simulink model "unfinished_Test_Display"  (Simulink 8.1)
settings: Solver=ode45  SolverMode=SingleTasking  StartTime=0.0  StopTime=2  RelTol=1e-3
undefined symbols (not defined in the file): A, ARROW_DOWN, ARROW_LEFT, ARROW_RIGHT, ARROW_UP, ASTERISK, B, BACKSLASH, C, COLON, COMMA, CROSS, CURSOR, D, DOT, EQUAL, EXCLAMATION_MARK, F, G, GREATER_THAN, H, HEIGHT, hot, I, J, K, L, LEFT_PARENTHESES, LESS_THAN, M, MINUS, N, O, P, PERCENT, PLUS, POS_X, POS_Y, Q, QUESTION_MARK, QUOTE, R, RECTANGLE, RIGHT_PARENTHESES, S, SEMICOLON, SHARP, SLASH, SPACE, T, U, UNDERSCORE, V, vect, W, WIDTH, X, Y, Z, ZERO
libraries: Common_Library x40, dspsnks4 x2, commutil2 x1
(part 2 of 3)

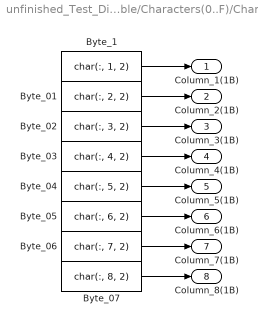
== system unfinished_Test_Display/Character_Table/Characters(0..F)/Char_2 ==
  Byte_01 : Constant  Value=char(:, 2, 2)  OutDataTypeStr=uint8
  Byte_02 : Constant  Value=char(:, 3, 2)  OutDataTypeStr=uint8
  Byte_03 : Constant  Value=char(:, 4, 2)  OutDataTypeStr=uint8
  Byte_04 : Constant  Value=char(:, 5, 2)  OutDataTypeStr=uint8
  Byte_05 : Constant  Value=char(:, 6, 2)  OutDataTypeStr=uint8
  Byte_06 : Constant  Value=char(:, 7, 2)  OutDataTypeStr=uint8
  Byte_07 : Constant  Value=char(:, 8, 2)  OutDataTypeStr=uint8
  Byte_1 : Constant  Value=char(:, 1, 2)  OutDataTypeStr=uint8
  Column_1(1B) : Outport
  Column_2(1B) : Outport  Port=2
  Column_3(1B) : Outport  Port=3
  Column_4(1B) : Outport  Port=4
  Column_5(1B) : Outport  Port=5
  Column_6(1B) : Outport  Port=6
  Column_7(1B) : Outport  Port=7
  Column_8(1B) : Outport  Port=8
  wires:
  Byte_05/1 -> Column_6(1B)/1
  Byte_04/1 -> Column_5(1B)/1
  Byte_01/1 -> Column_2(1B)/1
  Byte_07/1 -> Column_8(1B)/1
  Byte_03/1 -> Column_4(1B)/1
  Byte_06/1 -> Column_7(1B)/1
  Byte_1/1 -> Column_1(1B)/1
  Byte_02/1 -> Column_3(1B)/1

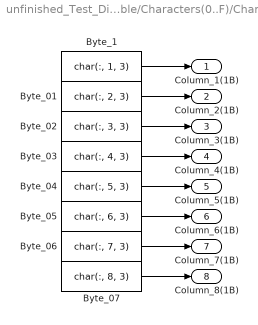
== system unfinished_Test_Display/Character_Table/Characters(0..F)/Char_3 ==
  Byte_01 : Constant  Value=char(:, 2, 3)  OutDataTypeStr=uint8
  Byte_02 : Constant  Value=char(:, 3, 3)  OutDataTypeStr=uint8
  Byte_03 : Constant  Value=char(:, 4, 3)  OutDataTypeStr=uint8
  Byte_04 : Constant  Value=char(:, 5, 3)  OutDataTypeStr=uint8
  Byte_05 : Constant  Value=char(:, 6, 3)  OutDataTypeStr=uint8
  Byte_06 : Constant  Value=char(:, 7, 3)  OutDataTypeStr=uint8
  Byte_07 : Constant  Value=char(:, 8, 3)  OutDataTypeStr=uint8
  Byte_1 : Constant  Value=char(:, 1, 3)  OutDataTypeStr=uint8
  Column_1(1B) : Outport
  Column_2(1B) : Outport  Port=2
  Column_3(1B) : Outport  Port=3
  Column_4(1B) : Outport  Port=4
  Column_5(1B) : Outport  Port=5
  Column_6(1B) : Outport  Port=6
  Column_7(1B) : Outport  Port=7
  Column_8(1B) : Outport  Port=8
  wires:
  Byte_05/1 -> Column_6(1B)/1
  Byte_04/1 -> Column_5(1B)/1
  Byte_01/1 -> Column_2(1B)/1
  Byte_07/1 -> Column_8(1B)/1
  Byte_03/1 -> Column_4(1B)/1
  Byte_06/1 -> Column_7(1B)/1
  Byte_1/1 -> Column_1(1B)/1
  Byte_02/1 -> Column_3(1B)/1

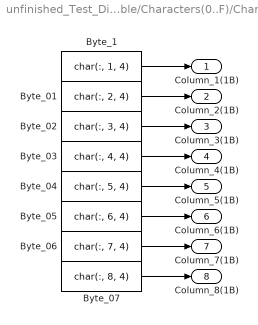
== system unfinished_Test_Display/Character_Table/Characters(0..F)/Char_4 ==
  Byte_01 : Constant  Value=char(:, 2, 4)  OutDataTypeStr=uint8
  Byte_02 : Constant  Value=char(:, 3, 4)  OutDataTypeStr=uint8
  Byte_03 : Constant  Value=char(:, 4, 4)  OutDataTypeStr=uint8
  Byte_04 : Constant  Value=char(:, 5, 4)  OutDataTypeStr=uint8
  Byte_05 : Constant  Value=char(:, 6, 4)  OutDataTypeStr=uint8
  Byte_06 : Constant  Value=char(:, 7, 4)  OutDataTypeStr=uint8
  Byte_07 : Constant  Value=char(:, 8, 4)  OutDataTypeStr=uint8
  Byte_1 : Constant  Value=char(:, 1, 4)  OutDataTypeStr=uint8
  Column_1(1B) : Outport
  Column_2(1B) : Outport  Port=2
  Column_3(1B) : Outport  Port=3
  Column_4(1B) : Outport  Port=4
  Column_5(1B) : Outport  Port=5
  Column_6(1B) : Outport  Port=6
  Column_7(1B) : Outport  Port=7
  Column_8(1B) : Outport  Port=8
  wires:
  Byte_05/1 -> Column_6(1B)/1
  Byte_04/1 -> Column_5(1B)/1
  Byte_01/1 -> Column_2(1B)/1
  Byte_07/1 -> Column_8(1B)/1
  Byte_03/1 -> Column_4(1B)/1
  Byte_06/1 -> Column_7(1B)/1
  Byte_1/1 -> Column_1(1B)/1
  Byte_02/1 -> Column_3(1B)/1

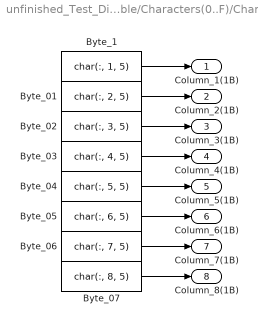
== system unfinished_Test_Display/Character_Table/Characters(0..F)/Char_5 ==
  Byte_01 : Constant  Value=char(:, 2, 5)  OutDataTypeStr=uint8
  Byte_02 : Constant  Value=char(:, 3, 5)  OutDataTypeStr=uint8
  Byte_03 : Constant  Value=char(:, 4, 5)  OutDataTypeStr=uint8
  Byte_04 : Constant  Value=char(:, 5, 5)  OutDataTypeStr=uint8
  Byte_05 : Constant  Value=char(:, 6, 5)  OutDataTypeStr=uint8
  Byte_06 : Constant  Value=char(:, 7, 5)  OutDataTypeStr=uint8
  Byte_07 : Constant  Value=char(:, 8, 5)  OutDataTypeStr=uint8
  Byte_1 : Constant  Value=char(:, 1, 5)  OutDataTypeStr=uint8
  Column_1(1B) : Outport
  Column_2(1B) : Outport  Port=2
  Column_3(1B) : Outport  Port=3
  Column_4(1B) : Outport  Port=4
  Column_5(1B) : Outport  Port=5
  Column_6(1B) : Outport  Port=6
  Column_7(1B) : Outport  Port=7
  Column_8(1B) : Outport  Port=8
  wires:
  Byte_05/1 -> Column_6(1B)/1
  Byte_04/1 -> Column_5(1B)/1
  Byte_01/1 -> Column_2(1B)/1
  Byte_07/1 -> Column_8(1B)/1
  Byte_03/1 -> Column_4(1B)/1
  Byte_06/1 -> Column_7(1B)/1
  Byte_1/1 -> Column_1(1B)/1
  Byte_02/1 -> Column_3(1B)/1

== system unfinished_Test_Display/Character_Table/Characters(0..F)/Char_6 ==
  Byte_01 : Constant  Value=char(:, 2, 6)  OutDataTypeStr=uint8
  Byte_02 : Constant  Value=char(:, 3, 6)  OutDataTypeStr=uint8
  Byte_03 : Constant  Value=char(:, 4, 6)  OutDataTypeStr=uint8
  Byte_04 : Constant  Value=char(:, 5, 6)  OutDataTypeStr=uint8
  Byte_05 : Constant  Value=char(:, 6, 6)  OutDataTypeStr=uint8
  Byte_06 : Constant  Value=char(:, 7, 6)  OutDataTypeStr=uint8
  Byte_07 : Constant  Value=char(:, 8, 6)  OutDataTypeStr=uint8
  Byte_1 : Constant  Value=char(:, 1, 6)  OutDataTypeStr=uint8
  Column_1(1B) : Outport
  Column_2(1B) : Outport  Port=2
  Column_3(1B) : Outport  Port=3
  Column_4(1B) : Outport  Port=4
  Column_5(1B) : Outport  Port=5
  Column_6(1B) : Outport  Port=6
  Column_7(1B) : Outport  Port=7
  Column_8(1B) : Outport  Port=8
  wires:
  Byte_05/1 -> Column_6(1B)/1
  Byte_04/1 -> Column_5(1B)/1
  Byte_01/1 -> Column_2(1B)/1
  Byte_07/1 -> Column_8(1B)/1
  Byte_03/1 -> Column_4(1B)/1
  Byte_06/1 -> Column_7(1B)/1
  Byte_1/1 -> Column_1(1B)/1
  Byte_02/1 -> Column_3(1B)/1

== system unfinished_Test_Display/Character_Table/Characters(0..F)/Char_7 ==
  Byte_01 : Constant  Value=char(:, 2, 7)  OutDataTypeStr=uint8
  Byte_02 : Constant  Value=char(:, 3, 7)  OutDataTypeStr=uint8
  Byte_03 : Constant  Value=char(:, 4, 7)  OutDataTypeStr=uint8
  Byte_04 : Constant  Value=char(:, 5, 7)  OutDataTypeStr=uint8
  Byte_05 : Constant  Value=char(:, 6, 7)  OutDataTypeStr=uint8
  Byte_06 : Constant  Value=char(:, 7, 7)  OutDataTypeStr=uint8
  Byte_07 : Constant  Value=char(:, 8, 7)  OutDataTypeStr=uint8
  Byte_1 : Constant  Value=char(:, 1, 7)  OutDataTypeStr=uint8
  Column_1(1B) : Outport
  Column_2(1B) : Outport  Port=2
  Column_3(1B) : Outport  Port=3
  Column_4(1B) : Outport  Port=4
  Column_5(1B) : Outport  Port=5
  Column_6(1B) : Outport  Port=6
  Column_7(1B) : Outport  Port=7
  Column_8(1B) : Outport  Port=8
  wires:
  Byte_05/1 -> Column_6(1B)/1
  Byte_04/1 -> Column_5(1B)/1
  Byte_01/1 -> Column_2(1B)/1
  Byte_07/1 -> Column_8(1B)/1
  Byte_03/1 -> Column_4(1B)/1
  Byte_06/1 -> Column_7(1B)/1
  Byte_1/1 -> Column_1(1B)/1
  Byte_02/1 -> Column_3(1B)/1

== system unfinished_Test_Display/Character_Table/Characters(0..F)/Char_8 ==
  Byte_01 : Constant  Value=char(:, 2, 8)  OutDataTypeStr=uint8
  Byte_02 : Constant  Value=char(:, 3, 8)  OutDataTypeStr=uint8
  Byte_03 : Constant  Value=char(:, 4, 8)  OutDataTypeStr=uint8
  Byte_04 : Constant  Value=char(:, 5, 8)  OutDataTypeStr=uint8
  Byte_05 : Constant  Value=char(:, 6, 8)  OutDataTypeStr=uint8
  Byte_06 : Constant  Value=char(:, 7, 8)  OutDataTypeStr=uint8
  Byte_07 : Constant  Value=char(:, 8, 8)  OutDataTypeStr=uint8
  Byte_1 : Constant  Value=char(:, 1, 8)  OutDataTypeStr=uint8
  Column_1(1B) : Outport
  Column_2(1B) : Outport  Port=2
  Column_3(1B) : Outport  Port=3
  Column_4(1B) : Outport  Port=4
  Column_5(1B) : Outport  Port=5
  Column_6(1B) : Outport  Port=6
  Column_7(1B) : Outport  Port=7
  Column_8(1B) : Outport  Port=8
  wires:
  Byte_05/1 -> Column_6(1B)/1
  Byte_04/1 -> Column_5(1B)/1
  Byte_01/1 -> Column_2(1B)/1
  Byte_07/1 -> Column_8(1B)/1
  Byte_03/1 -> Column_4(1B)/1
  Byte_06/1 -> Column_7(1B)/1
  Byte_1/1 -> Column_1(1B)/1
  Byte_02/1 -> Column_3(1B)/1

== system unfinished_Test_Display/Character_Table/Characters(0..F)/Char_9 ==
  Byte_01 : Constant  Value=char(:, 2, 9)  OutDataTypeStr=uint8
  Byte_02 : Constant  Value=char(:, 3, 9)  OutDataTypeStr=uint8
  Byte_03 : Constant  Value=char(:, 4, 9)  OutDataTypeStr=uint8
  Byte_04 : Constant  Value=char(:, 5, 9)  OutDataTypeStr=uint8
  Byte_05 : Constant  Value=char(:, 6, 9)  OutDataTypeStr=uint8
  Byte_06 : Constant  Value=char(:, 7, 9)  OutDataTypeStr=uint8
  Byte_07 : Constant  Value=char(:, 8, 9)  OutDataTypeStr=uint8
  Byte_1 : Constant  Value=char(:, 1, 9)  OutDataTypeStr=uint8
  Column_1(1B) : Outport
  Column_2(1B) : Outport  Port=2
  Column_3(1B) : Outport  Port=3
  Column_4(1B) : Outport  Port=4
  Column_5(1B) : Outport  Port=5
  Column_6(1B) : Outport  Port=6
  Column_7(1B) : Outport  Port=7
  Column_8(1B) : Outport  Port=8
  wires:
  Byte_05/1 -> Column_6(1B)/1
  Byte_04/1 -> Column_5(1B)/1
  Byte_01/1 -> Column_2(1B)/1
  Byte_07/1 -> Column_8(1B)/1
  Byte_03/1 -> Column_4(1B)/1
  Byte_06/1 -> Column_7(1B)/1
  Byte_1/1 -> Column_1(1B)/1
  Byte_02/1 -> Column_3(1B)/1

== system unfinished_Test_Display/Character_Table/Characters(0..F)/Char_A ==
  Byte_01 : Constant  Value=char(:, 2, A)  OutDataTypeStr=uint8
  Byte_02 : Constant  Value=char(:, 3, A)  OutDataTypeStr=uint8
  Byte_03 : Constant  Value=char(:, 4, A)  OutDataTypeStr=uint8
  Byte_04 : Constant  Value=char(:, 5, A)  OutDataTypeStr=uint8
  Byte_05 : Constant  Value=char(:, 6, A)  OutDataTypeStr=uint8
  Byte_06 : Constant  Value=char(:, 7, A)  OutDataTypeStr=uint8
  Byte_07 : Constant  Value=char(:, 8, A)  OutDataTypeStr=uint8
  Byte_1 : Constant  Value=char(:, 1, A)  OutDataTypeStr=uint8
  Column_1(1B) : Outport
  Column_2(1B) : Outport  Port=2
  Column_3(1B) : Outport  Port=3
  Column_4(1B) : Outport  Port=4
  Column_5(1B) : Outport  Port=5
  Column_6(1B) : Outport  Port=6
  Column_7(1B) : Outport  Port=7
  Column_8(1B) : Outport  Port=8
  wires:
  Byte_05/1 -> Column_6(1B)/1
  Byte_04/1 -> Column_5(1B)/1
  Byte_01/1 -> Column_2(1B)/1
  Byte_07/1 -> Column_8(1B)/1
  Byte_03/1 -> Column_4(1B)/1
  Byte_06/1 -> Column_7(1B)/1
  Byte_1/1 -> Column_1(1B)/1
  Byte_02/1 -> Column_3(1B)/1

== system unfinished_Test_Display/Character_Table/Characters(0..F)/Char_B ==
  Byte_01 : Constant  Value=char(:, 2, B)  OutDataTypeStr=uint8
  Byte_02 : Constant  Value=char(:, 3, B)  OutDataTypeStr=uint8
  Byte_03 : Constant  Value=char(:, 4, B)  OutDataTypeStr=uint8
  Byte_04 : Constant  Value=char(:, 5, B)  OutDataTypeStr=uint8
  Byte_05 : Constant  Value=char(:, 6, B)  OutDataTypeStr=uint8
  Byte_06 : Constant  Value=char(:, 7, B)  OutDataTypeStr=uint8
  Byte_07 : Constant  Value=char(:, 8, B)  OutDataTypeStr=uint8
  Byte_1 : Constant  Value=char(:, 1, B)  OutDataTypeStr=uint8
  Column_1(1B) : Outport
  Column_2(1B) : Outport  Port=2
  Column_3(1B) : Outport  Port=3
  Column_4(1B) : Outport  Port=4
  Column_5(1B) : Outport  Port=5
  Column_6(1B) : Outport  Port=6
  Column_7(1B) : Outport  Port=7
  Column_8(1B) : Outport  Port=8
  wires:
  Byte_05/1 -> Column_6(1B)/1
  Byte_04/1 -> Column_5(1B)/1
  Byte_01/1 -> Column_2(1B)/1
  Byte_07/1 -> Column_8(1B)/1
  Byte_03/1 -> Column_4(1B)/1
  Byte_06/1 -> Column_7(1B)/1
  Byte_1/1 -> Column_1(1B)/1
  Byte_02/1 -> Column_3(1B)/1

== system unfinished_Test_Display/Character_Table/Characters(0..F)/Char_C ==
  Byte_01 : Constant  Value=char(:, 2, C)  OutDataTypeStr=uint8
  Byte_02 : Constant  Value=char(:, 3, C)  OutDataTypeStr=uint8
  Byte_03 : Constant  Value=char(:, 4, C)  OutDataTypeStr=uint8
  Byte_04 : Constant  Value=char(:, 5, C)  OutDataTypeStr=uint8
  Byte_05 : Constant  Value=char(:, 6, C)  OutDataTypeStr=uint8
  Byte_06 : Constant  Value=char(:, 7, C)  OutDataTypeStr=uint8
  Byte_07 : Constant  Value=char(:, 8, C)  OutDataTypeStr=uint8
  Byte_1 : Constant  Value=char(:, 1, C)  OutDataTypeStr=uint8
  Column_1(1B) : Outport
  Column_2(1B) : Outport  Port=2
  Column_3(1B) : Outport  Port=3
  Column_4(1B) : Outport  Port=4
  Column_5(1B) : Outport  Port=5
  Column_6(1B) : Outport  Port=6
  Column_7(1B) : Outport  Port=7
  Column_8(1B) : Outport  Port=8
  wires:
  Byte_05/1 -> Column_6(1B)/1
  Byte_04/1 -> Column_5(1B)/1
  Byte_01/1 -> Column_2(1B)/1
  Byte_07/1 -> Column_8(1B)/1
  Byte_03/1 -> Column_4(1B)/1
  Byte_06/1 -> Column_7(1B)/1
  Byte_1/1 -> Column_1(1B)/1
  Byte_02/1 -> Column_3(1B)/1

== system unfinished_Test_Display/Character_Table/Characters(0..F)/Char_D ==
  Byte_01 : Constant  Value=char(:, 2, D)  OutDataTypeStr=uint8
  Byte_02 : Constant  Value=char(:, 3, D)  OutDataTypeStr=uint8
  Byte_03 : Constant  Value=char(:, 4, D)  OutDataTypeStr=uint8
  Byte_04 : Constant  Value=char(:, 5, D)  OutDataTypeStr=uint8
  Byte_05 : Constant  Value=char(:, 6, D)  OutDataTypeStr=uint8
  Byte_06 : Constant  Value=char(:, 7, D)  OutDataTypeStr=uint8
  Byte_07 : Constant  Value=char(:, 8, D)  OutDataTypeStr=uint8
  Byte_1 : Constant  Value=char(:, 1, D)  OutDataTypeStr=uint8
  Column_1(1B) : Outport
  Column_2(1B) : Outport  Port=2
  Column_3(1B) : Outport  Port=3
  Column_4(1B) : Outport  Port=4
  Column_5(1B) : Outport  Port=5
  Column_6(1B) : Outport  Port=6
  Column_7(1B) : Outport  Port=7
  Column_8(1B) : Outport  Port=8
  wires:
  Byte_05/1 -> Column_6(1B)/1
  Byte_04/1 -> Column_5(1B)/1
  Byte_01/1 -> Column_2(1B)/1
  Byte_07/1 -> Column_8(1B)/1
  Byte_03/1 -> Column_4(1B)/1
  Byte_06/1 -> Column_7(1B)/1
  Byte_1/1 -> Column_1(1B)/1
  Byte_02/1 -> Column_3(1B)/1

== system unfinished_Test_Display/Character_Table/Characters(0..F)/Char_E ==
  Byte_01 : Constant  Value=char(:, 2, E)  OutDataTypeStr=uint8
  Byte_02 : Constant  Value=char(:, 3, E)  OutDataTypeStr=uint8
  Byte_03 : Constant  Value=char(:, 4, E)  OutDataTypeStr=uint8
  Byte_04 : Constant  Value=char(:, 5, E)  OutDataTypeStr=uint8
  Byte_05 : Constant  Value=char(:, 6, E)  OutDataTypeStr=uint8
  Byte_06 : Constant  Value=char(:, 7, E)  OutDataTypeStr=uint8
  Byte_07 : Constant  Value=char(:, 8, E)  OutDataTypeStr=uint8
  Byte_1 : Constant  Value=char(:, 1, E)  OutDataTypeStr=uint8
  Column_1(1B) : Outport
  Column_2(1B) : Outport  Port=2
  Column_3(1B) : Outport  Port=3
  Column_4(1B) : Outport  Port=4
  Column_5(1B) : Outport  Port=5
  Column_6(1B) : Outport  Port=6
  Column_7(1B) : Outport  Port=7
  Column_8(1B) : Outport  Port=8
  wires:
  Byte_05/1 -> Column_6(1B)/1
  Byte_04/1 -> Column_5(1B)/1
  Byte_01/1 -> Column_2(1B)/1
  Byte_07/1 -> Column_8(1B)/1
  Byte_03/1 -> Column_4(1B)/1
  Byte_06/1 -> Column_7(1B)/1
  Byte_1/1 -> Column_1(1B)/1
  Byte_02/1 -> Column_3(1B)/1

== system unfinished_Test_Display/Character_Table/Characters(0..F)/Char_F ==
  Byte_01 : Constant  Value=char(:, 2, F)  OutDataTypeStr=uint8
  Byte_02 : Constant  Value=char(:, 3, F)  OutDataTypeStr=uint8
  Byte_03 : Constant  Value=char(:, 4, F)  OutDataTypeStr=uint8
  Byte_04 : Constant  Value=char(:, 5, F)  OutDataTypeStr=uint8
  Byte_05 : Constant  Value=char(:, 6, F)  OutDataTypeStr=uint8
  Byte_06 : Constant  Value=char(:, 7, F)  OutDataTypeStr=uint8
  Byte_07 : Constant  Value=char(:, 8, F)  OutDataTypeStr=uint8
  Byte_1 : Constant  Value=char(:, 1, F)  OutDataTypeStr=uint8
  Column_1(1B) : Outport
  Column_2(1B) : Outport  Port=2
  Column_3(1B) : Outport  Port=3
  Column_4(1B) : Outport  Port=4
  Column_5(1B) : Outport  Port=5
  Column_6(1B) : Outport  Port=6
  Column_7(1B) : Outport  Port=7
  Column_8(1B) : Outport  Port=8
  wires:
  Byte_05/1 -> Column_6(1B)/1
  Byte_04/1 -> Column_5(1B)/1
  Byte_01/1 -> Column_2(1B)/1
  Byte_07/1 -> Column_8(1B)/1
  Byte_03/1 -> Column_4(1B)/1
  Byte_06/1 -> Column_7(1B)/1
  Byte_1/1 -> Column_1(1B)/1
  Byte_02/1 -> Column_3(1B)/1

== system unfinished_Test_Display/Character_Table/Characters(ARROW_DOWN..RECTANGLE)/Char_ARROW_DOWN ==
  Byte_01 : Constant  Value=char(:, 2, ARROW_DOWN)  OutDataTypeStr=uint8
  Byte_02 : Constant  Value=char(:, 3, ARROW_DOWN)  OutDataTypeStr=uint8
  Byte_03 : Constant  Value=char(:, 4, ARROW_DOWN)  OutDataTypeStr=uint8
  Byte_04 : Constant  Value=char(:, 5, ARROW_DOWN)  OutDataTypeStr=uint8
  Byte_05 : Constant  Value=char(:, 6, ARROW_DOWN)  OutDataTypeStr=uint8
  Byte_06 : Constant  Value=char(:, 7, ARROW_DOWN)  OutDataTypeStr=uint8
  Byte_07 : Constant  Value=char(:, 8, ARROW_DOWN)  OutDataTypeStr=uint8
  Byte_1 : Constant  Value=char(:, 1, ARROW_DOWN)  OutDataTypeStr=uint8
  Column_1(1B) : Outport
  Column_2(1B) : Outport  Port=2
  Column_3(1B) : Outport  Port=3
  Column_4(1B) : Outport  Port=4
  Column_5(1B) : Outport  Port=5
  Column_6(1B) : Outport  Port=6
  Column_7(1B) : Outport  Port=7
  Column_8(1B) : Outport  Port=8
  wires:
  Byte_05/1 -> Column_6(1B)/1
  Byte_04/1 -> Column_5(1B)/1
  Byte_01/1 -> Column_2(1B)/1
  Byte_07/1 -> Column_8(1B)/1
  Byte_03/1 -> Column_4(1B)/1
  Byte_06/1 -> Column_7(1B)/1
  Byte_1/1 -> Column_1(1B)/1
  Byte_02/1 -> Column_3(1B)/1

== system unfinished_Test_Display/Character_Table/Characters(ARROW_DOWN..RECTANGLE)/Char_ARROW_LEFT ==
  Byte_01 : Constant  Value=char(:, 2, ARROW_LEFT)  OutDataTypeStr=uint8
  Byte_02 : Constant  Value=char(:, 3, ARROW_LEFT)  OutDataTypeStr=uint8
  Byte_03 : Constant  Value=char(:, 4, ARROW_LEFT)  OutDataTypeStr=uint8
  Byte_04 : Constant  Value=char(:, 5, ARROW_LEFT)  OutDataTypeStr=uint8
  Byte_05 : Constant  Value=char(:, 6, ARROW_LEFT)  OutDataTypeStr=uint8
  Byte_06 : Constant  Value=char(:, 7, ARROW_LEFT)  OutDataTypeStr=uint8
  Byte_07 : Constant  Value=char(:, 8, ARROW_LEFT)  OutDataTypeStr=uint8
  Byte_1 : Constant  Value=char(:, 1, ARROW_LEFT)  OutDataTypeStr=uint8
  Column_1(1B) : Outport
  Column_2(1B) : Outport  Port=2
  Column_3(1B) : Outport  Port=3
  Column_4(1B) : Outport  Port=4
  Column_5(1B) : Outport  Port=5
  Column_6(1B) : Outport  Port=6
  Column_7(1B) : Outport  Port=7
  Column_8(1B) : Outport  Port=8
  wires:
  Byte_05/1 -> Column_6(1B)/1
  Byte_04/1 -> Column_5(1B)/1
  Byte_01/1 -> Column_2(1B)/1
  Byte_07/1 -> Column_8(1B)/1
  Byte_03/1 -> Column_4(1B)/1
  Byte_06/1 -> Column_7(1B)/1
  Byte_1/1 -> Column_1(1B)/1
  Byte_02/1 -> Column_3(1B)/1

== system unfinished_Test_Display/Character_Table/Characters(ARROW_DOWN..RECTANGLE)/Char_ARROW_RIGHT ==
  Byte_01 : Constant  Value=char(:, 2, ARROW_RIGHT)  OutDataTypeStr=uint8
  Byte_02 : Constant  Value=char(:, 3, ARROW_RIGHT)  OutDataTypeStr=uint8
  Byte_03 : Constant  Value=char(:, 4, ARROW_RIGHT)  OutDataTypeStr=uint8
  Byte_04 : Constant  Value=char(:, 5, ARROW_RIGHT)  OutDataTypeStr=uint8
  Byte_05 : Constant  Value=char(:, 6, ARROW_RIGHT)  OutDataTypeStr=uint8
  Byte_06 : Constant  Value=char(:, 7, ARROW_RIGHT)  OutDataTypeStr=uint8
  Byte_07 : Constant  Value=char(:, 8, ARROW_RIGHT)  OutDataTypeStr=uint8
  Byte_1 : Constant  Value=char(:, 1, ARROW_RIGHT)  OutDataTypeStr=uint8
  Column_1(1B) : Outport
  Column_2(1B) : Outport  Port=2
  Column_3(1B) : Outport  Port=3
  Column_4(1B) : Outport  Port=4
  Column_5(1B) : Outport  Port=5
  Column_6(1B) : Outport  Port=6
  Column_7(1B) : Outport  Port=7
  Column_8(1B) : Outport  Port=8
  wires:
  Byte_05/1 -> Column_6(1B)/1
  Byte_04/1 -> Column_5(1B)/1
  Byte_01/1 -> Column_2(1B)/1
  Byte_07/1 -> Column_8(1B)/1
  Byte_03/1 -> Column_4(1B)/1
  Byte_06/1 -> Column_7(1B)/1
  Byte_1/1 -> Column_1(1B)/1
  Byte_02/1 -> Column_3(1B)/1

== system unfinished_Test_Display/Character_Table/Characters(ARROW_DOWN..RECTANGLE)/Char_COMMA ==
  Byte_01 : Constant  Value=char(:, 2, COMMA)  OutDataTypeStr=uint8
  Byte_02 : Constant  Value=char(:, 3, COMMA)  OutDataTypeStr=uint8
  Byte_03 : Constant  Value=char(:, 4, COMMA)  OutDataTypeStr=uint8
  Byte_04 : Constant  Value=char(:, 5, COMMA)  OutDataTypeStr=uint8
  Byte_05 : Constant  Value=char(:, 6, COMMA)  OutDataTypeStr=uint8
  Byte_06 : Constant  Value=char(:, 7, COMMA)  OutDataTypeStr=uint8
  Byte_07 : Constant  Value=char(:, 8, COMMA)  OutDataTypeStr=uint8
  Byte_1 : Constant  Value=char(:, 1, COMMA)  OutDataTypeStr=uint8
  Column_1(1B) : Outport
  Column_2(1B) : Outport  Port=2
  Column_3(1B) : Outport  Port=3
  Column_4(1B) : Outport  Port=4
  Column_5(1B) : Outport  Port=5
  Column_6(1B) : Outport  Port=6
  Column_7(1B) : Outport  Port=7
  Column_8(1B) : Outport  Port=8
  wires:
  Byte_05/1 -> Column_6(1B)/1
  Byte_04/1 -> Column_5(1B)/1
  Byte_01/1 -> Column_2(1B)/1
  Byte_07/1 -> Column_8(1B)/1
  Byte_03/1 -> Column_4(1B)/1
  Byte_06/1 -> Column_7(1B)/1
  Byte_1/1 -> Column_1(1B)/1
  Byte_02/1 -> Column_3(1B)/1

== system unfinished_Test_Display/Character_Table/Characters(ARROW_DOWN..RECTANGLE)/Char_CURSOR ==
  Byte_01 : Constant  Value=char(:, 2, CURSOR)  OutDataTypeStr=uint8
  Byte_02 : Constant  Value=char(:, 3, CURSOR)  OutDataTypeStr=uint8
  Byte_03 : Constant  Value=char(:, 4, CURSOR)  OutDataTypeStr=uint8
  Byte_04 : Constant  Value=char(:, 5, CURSOR)  OutDataTypeStr=uint8
  Byte_05 : Constant  Value=char(:, 6, CURSOR)  OutDataTypeStr=uint8
  Byte_06 : Constant  Value=char(:, 7, CURSOR)  OutDataTypeStr=uint8
  Byte_07 : Constant  Value=char(:, 8, CURSOR)  OutDataTypeStr=uint8
  Byte_1 : Constant  Value=char(:, 1, CURSOR)  OutDataTypeStr=uint8
  Column_1(1B) : Outport
  Column_2(1B) : Outport  Port=2
  Column_3(1B) : Outport  Port=3
  Column_4(1B) : Outport  Port=4
  Column_5(1B) : Outport  Port=5
  Column_6(1B) : Outport  Port=6
  Column_7(1B) : Outport  Port=7
  Column_8(1B) : Outport  Port=8
  wires:
  Byte_05/1 -> Column_6(1B)/1
  Byte_04/1 -> Column_5(1B)/1
  Byte_01/1 -> Column_2(1B)/1
  Byte_07/1 -> Column_8(1B)/1
  Byte_03/1 -> Column_4(1B)/1
  Byte_06/1 -> Column_7(1B)/1
  Byte_1/1 -> Column_1(1B)/1
  Byte_02/1 -> Column_3(1B)/1

== system unfinished_Test_Display/Character_Table/Characters(ARROW_DOWN..RECTANGLE)/Char_DOT ==
  Byte_01 : Constant  Value=char(:, 2, DOT)  OutDataTypeStr=uint8
  Byte_02 : Constant  Value=char(:, 3, DOT)  OutDataTypeStr=uint8
  Byte_03 : Constant  Value=char(:, 4, DOT)  OutDataTypeStr=uint8
  Byte_04 : Constant  Value=char(:, 5, DOT)  OutDataTypeStr=uint8
  Byte_05 : Constant  Value=char(:, 6, DOT)  OutDataTypeStr=uint8
  Byte_06 : Constant  Value=char(:, 7, DOT)  OutDataTypeStr=uint8
  Byte_07 : Constant  Value=char(:, 8, DOT)  OutDataTypeStr=uint8
  Byte_1 : Constant  Value=char(:, 1, DOT)  OutDataTypeStr=uint8
  Column_1(1B) : Outport
  Column_2(1B) : Outport  Port=2
  Column_3(1B) : Outport  Port=3
  Column_4(1B) : Outport  Port=4
  Column_5(1B) : Outport  Port=5
  Column_6(1B) : Outport  Port=6
  Column_7(1B) : Outport  Port=7
  Column_8(1B) : Outport  Port=8
  wires:
  Byte_05/1 -> Column_6(1B)/1
  Byte_04/1 -> Column_5(1B)/1
  Byte_01/1 -> Column_2(1B)/1
  Byte_07/1 -> Column_8(1B)/1
  Byte_03/1 -> Column_4(1B)/1
  Byte_06/1 -> Column_7(1B)/1
  Byte_1/1 -> Column_1(1B)/1
  Byte_02/1 -> Column_3(1B)/1

== system unfinished_Test_Display/Character_Table/Characters(ARROW_DOWN..RECTANGLE)/Char_EXCLAMATION_MARK ==
  Byte_01 : Constant  Value=char(:, 2, EXCLAMATION_MARK)  OutDataTypeStr=uint8
  Byte_02 : Constant  Value=char(:, 3, EXCLAMATION_MARK)  OutDataTypeStr=uint8
  Byte_03 : Constant  Value=char(:, 4, EXCLAMATION_MARK)  OutDataTypeStr=uint8
  Byte_04 : Constant  Value=char(:, 5, EXCLAMATION_MARK)  OutDataTypeStr=uint8
  Byte_05 : Constant  Value=char(:, 6, EXCLAMATION_MARK)  OutDataTypeStr=uint8
  Byte_06 : Constant  Value=char(:, 7, EXCLAMATION_MARK)  OutDataTypeStr=uint8
  Byte_07 : Constant  Value=char(:, 8, EXCLAMATION_MARK)  OutDataTypeStr=uint8
  Byte_1 : Constant  Value=char(:, 1, EXCLAMATION_MARK)  OutDataTypeStr=uint8
  Column_1(1B) : Outport
  Column_2(1B) : Outport  Port=2
  Column_3(1B) : Outport  Port=3
  Column_4(1B) : Outport  Port=4
  Column_5(1B) : Outport  Port=5
  Column_6(1B) : Outport  Port=6
  Column_7(1B) : Outport  Port=7
  Column_8(1B) : Outport  Port=8
  wires:
  Byte_05/1 -> Column_6(1B)/1
  Byte_04/1 -> Column_5(1B)/1
  Byte_01/1 -> Column_2(1B)/1
  Byte_07/1 -> Column_8(1B)/1
  Byte_03/1 -> Column_4(1B)/1
  Byte_06/1 -> Column_7(1B)/1
  Byte_1/1 -> Column_1(1B)/1
  Byte_02/1 -> Column_3(1B)/1

== system unfinished_Test_Display/Character_Table/Characters(ARROW_DOWN..RECTANGLE)/Char_LEFT_PARENTHESES ==
  Byte_01 : Constant  Value=char(:, 2, LEFT_PARENTHESES)  OutDataTypeStr=uint8
  Byte_02 : Constant  Value=char(:, 3, LEFT_PARENTHESES)  OutDataTypeStr=uint8
  Byte_03 : Constant  Value=char(:, 4, LEFT_PARENTHESES)  OutDataTypeStr=uint8
  Byte_04 : Constant  Value=char(:, 5, LEFT_PARENTHESES)  OutDataTypeStr=uint8
  Byte_05 : Constant  Value=char(:, 6, LEFT_PARENTHESES)  OutDataTypeStr=uint8
  Byte_06 : Constant  Value=char(:, 7, LEFT_PARENTHESES)  OutDataTypeStr=uint8
  Byte_07 : Constant  Value=char(:, 8, LEFT_PARENTHESES)  OutDataTypeStr=uint8
  Byte_1 : Constant  Value=char(:, 1, LEFT_PARENTHESES)  OutDataTypeStr=uint8
  Column_1(1B) : Outport
  Column_2(1B) : Outport  Port=2
  Column_3(1B) : Outport  Port=3
  Column_4(1B) : Outport  Port=4
  Column_5(1B) : Outport  Port=5
  Column_6(1B) : Outport  Port=6
  Column_7(1B) : Outport  Port=7
  Column_8(1B) : Outport  Port=8
  wires:
  Byte_05/1 -> Column_6(1B)/1
  Byte_04/1 -> Column_5(1B)/1
  Byte_01/1 -> Column_2(1B)/1
  Byte_07/1 -> Column_8(1B)/1
  Byte_03/1 -> Column_4(1B)/1
  Byte_06/1 -> Column_7(1B)/1
  Byte_1/1 -> Column_1(1B)/1
  Byte_02/1 -> Column_3(1B)/1

== system unfinished_Test_Display/Character_Table/Characters(ARROW_DOWN..RECTANGLE)/Char_PERCENT ==
  Byte_01 : Constant  Value=char(:, 2, PERCENT)  OutDataTypeStr=uint8
  Byte_02 : Constant  Value=char(:, 3, PERCENT)  OutDataTypeStr=uint8
  Byte_03 : Constant  Value=char(:, 4, PERCENT)  OutDataTypeStr=uint8
  Byte_04 : Constant  Value=char(:, 5, PERCENT)  OutDataTypeStr=uint8
  Byte_05 : Constant  Value=char(:, 6, PERCENT)  OutDataTypeStr=uint8
  Byte_06 : Constant  Value=char(:, 7, PERCENT)  OutDataTypeStr=uint8
  Byte_07 : Constant  Value=char(:, 8, PERCENT)  OutDataTypeStr=uint8
  Byte_1 : Constant  Value=char(:, 1, PERCENT)  OutDataTypeStr=uint8
  Column_1(1B) : Outport
  Column_2(1B) : Outport  Port=2
  Column_3(1B) : Outport  Port=3
  Column_4(1B) : Outport  Port=4
  Column_5(1B) : Outport  Port=5
  Column_6(1B) : Outport  Port=6
  Column_7(1B) : Outport  Port=7
  Column_8(1B) : Outport  Port=8
  wires:
  Byte_05/1 -> Column_6(1B)/1
  Byte_04/1 -> Column_5(1B)/1
  Byte_01/1 -> Column_2(1B)/1
  Byte_07/1 -> Column_8(1B)/1
  Byte_03/1 -> Column_4(1B)/1
  Byte_06/1 -> Column_7(1B)/1
  Byte_1/1 -> Column_1(1B)/1
  Byte_02/1 -> Column_3(1B)/1

== system unfinished_Test_Display/Character_Table/Characters(ARROW_DOWN..RECTANGLE)/Char_QUESTION_MARK ==
  Byte_01 : Constant  Value=char(:, 2, QUESTION_MARK)  OutDataTypeStr=uint8
  Byte_02 : Constant  Value=char(:, 3, QUESTION_MARK)  OutDataTypeStr=uint8
  Byte_03 : Constant  Value=char(:, 4, QUESTION_MARK)  OutDataTypeStr=uint8
  Byte_04 : Constant  Value=char(:, 5, QUESTION_MARK)  OutDataTypeStr=uint8
  Byte_05 : Constant  Value=char(:, 6, QUESTION_MARK)  OutDataTypeStr=uint8
  Byte_06 : Constant  Value=char(:, 7, QUESTION_MARK)  OutDataTypeStr=uint8
  Byte_07 : Constant  Value=char(:, 8, QUESTION_MARK)  OutDataTypeStr=uint8
  Byte_1 : Constant  Value=char(:, 1, QUESTION_MARK)  OutDataTypeStr=uint8
  Column_1(1B) : Outport
  Column_2(1B) : Outport  Port=2
  Column_3(1B) : Outport  Port=3
  Column_4(1B) : Outport  Port=4
  Column_5(1B) : Outport  Port=5
  Column_6(1B) : Outport  Port=6
  Column_7(1B) : Outport  Port=7
  Column_8(1B) : Outport  Port=8
  wires:
  Byte_05/1 -> Column_6(1B)/1
  Byte_04/1 -> Column_5(1B)/1
  Byte_01/1 -> Column_2(1B)/1
  Byte_07/1 -> Column_8(1B)/1
  Byte_03/1 -> Column_4(1B)/1
  Byte_06/1 -> Column_7(1B)/1
  Byte_1/1 -> Column_1(1B)/1
  Byte_02/1 -> Column_3(1B)/1

== system unfinished_Test_Display/Character_Table/Characters(ARROW_DOWN..RECTANGLE)/Char_QUOTE ==
  Byte_01 : Constant  Value=char(:, 2, QUOTE)  OutDataTypeStr=uint8
  Byte_02 : Constant  Value=char(:, 3, QUOTE)  OutDataTypeStr=uint8
  Byte_03 : Constant  Value=char(:, 4, QUOTE)  OutDataTypeStr=uint8
  Byte_04 : Constant  Value=char(:, 5, QUOTE)  OutDataTypeStr=uint8
  Byte_05 : Constant  Value=char(:, 6, QUOTE)  OutDataTypeStr=uint8
  Byte_06 : Constant  Value=char(:, 7, QUOTE)  OutDataTypeStr=uint8
  Byte_07 : Constant  Value=char(:, 8, QUOTE)  OutDataTypeStr=uint8
  Byte_1 : Constant  Value=char(:, 1, QUOTE)  OutDataTypeStr=uint8
  Column_1(1B) : Outport
  Column_2(1B) : Outport  Port=2
  Column_3(1B) : Outport  Port=3
  Column_4(1B) : Outport  Port=4
  Column_5(1B) : Outport  Port=5
  Column_6(1B) : Outport  Port=6
  Column_7(1B) : Outport  Port=7
  Column_8(1B) : Outport  Port=8
  wires:
  Byte_05/1 -> Column_6(1B)/1
  Byte_04/1 -> Column_5(1B)/1
  Byte_01/1 -> Column_2(1B)/1
  Byte_07/1 -> Column_8(1B)/1
  Byte_03/1 -> Column_4(1B)/1
  Byte_06/1 -> Column_7(1B)/1
  Byte_1/1 -> Column_1(1B)/1
  Byte_02/1 -> Column_3(1B)/1

== system unfinished_Test_Display/Character_Table/Characters(ARROW_DOWN..RECTANGLE)/Char_RECTANGLE ==
  Byte_01 : Constant  Value=char(:, 2, RECTANGLE)  OutDataTypeStr=uint8
  Byte_02 : Constant  Value=char(:, 3, RECTANGLE)  OutDataTypeStr=uint8
  Byte_03 : Constant  Value=char(:, 4, RECTANGLE)  OutDataTypeStr=uint8
  Byte_04 : Constant  Value=char(:, 5, RECTANGLE)  OutDataTypeStr=uint8
  Byte_05 : Constant  Value=char(:, 6, RECTANGLE)  OutDataTypeStr=uint8
  Byte_06 : Constant  Value=char(:, 7, RECTANGLE)  OutDataTypeStr=uint8
  Byte_07 : Constant  Value=char(:, 8, RECTANGLE)  OutDataTypeStr=uint8
  Byte_1 : Constant  Value=char(:, 1, RECTANGLE)  OutDataTypeStr=uint8
  Column_1(1B) : Outport
  Column_2(1B) : Outport  Port=2
  Column_3(1B) : Outport  Port=3
  Column_4(1B) : Outport  Port=4
  Column_5(1B) : Outport  Port=5
  Column_6(1B) : Outport  Port=6
  Column_7(1B) : Outport  Port=7
  Column_8(1B) : Outport  Port=8
  wires:
  Byte_05/1 -> Column_6(1B)/1
  Byte_04/1 -> Column_5(1B)/1
  Byte_01/1 -> Column_2(1B)/1
  Byte_07/1 -> Column_8(1B)/1
  Byte_03/1 -> Column_4(1B)/1
  Byte_06/1 -> Column_7(1B)/1
  Byte_1/1 -> Column_1(1B)/1
  Byte_02/1 -> Column_3(1B)/1

== system unfinished_Test_Display/Character_Table/Characters(ARROW_DOWN..RECTANGLE)/Char_RIGHT_PARENTHESES ==
  Byte_01 : Constant  Value=char(:, 2, RIGHT_PARENTHESES)  OutDataTypeStr=uint8
  Byte_02 : Constant  Value=char(:, 3, RIGHT_PARENTHESES)  OutDataTypeStr=uint8
  Byte_03 : Constant  Value=char(:, 4, RIGHT_PARENTHESES)  OutDataTypeStr=uint8
  Byte_04 : Constant  Value=char(:, 5, RIGHT_PARENTHESES)  OutDataTypeStr=uint8
  Byte_05 : Constant  Value=char(:, 6, RIGHT_PARENTHESES)  OutDataTypeStr=uint8
  Byte_06 : Constant  Value=char(:, 7, RIGHT_PARENTHESES)  OutDataTypeStr=uint8
  Byte_07 : Constant  Value=char(:, 8, RIGHT_PARENTHESES)  OutDataTypeStr=uint8
  Byte_1 : Constant  Value=char(:, 1, RIGHT_PARENTHESES)  OutDataTypeStr=uint8
  Column_1(1B) : Outport
  Column_2(1B) : Outport  Port=2
  Column_3(1B) : Outport  Port=3
  Column_4(1B) : Outport  Port=4
  Column_5(1B) : Outport  Port=5
  Column_6(1B) : Outport  Port=6
  Column_7(1B) : Outport  Port=7
  Column_8(1B) : Outport  Port=8
  wires:
  Byte_05/1 -> Column_6(1B)/1
  Byte_04/1 -> Column_5(1B)/1
  Byte_01/1 -> Column_2(1B)/1
  Byte_07/1 -> Column_8(1B)/1
  Byte_03/1 -> Column_4(1B)/1
  Byte_06/1 -> Column_7(1B)/1
  Byte_1/1 -> Column_1(1B)/1
  Byte_02/1 -> Column_3(1B)/1

== system unfinished_Test_Display/Character_Table/Characters(ARROW_DOWN..RECTANGLE)/Char_SHARP ==
  Byte_01 : Constant  Value=char(:, 2, SHARP)  OutDataTypeStr=uint8
  Byte_02 : Constant  Value=char(:, 3, SHARP)  OutDataTypeStr=uint8
  Byte_03 : Constant  Value=char(:, 4, SHARP)  OutDataTypeStr=uint8
  Byte_04 : Constant  Value=char(:, 5, SHARP)  OutDataTypeStr=uint8
  Byte_05 : Constant  Value=char(:, 6, SHARP)  OutDataTypeStr=uint8
  Byte_06 : Constant  Value=char(:, 7, SHARP)  OutDataTypeStr=uint8
  Byte_07 : Constant  Value=char(:, 8, SHARP)  OutDataTypeStr=uint8
  Byte_1 : Constant  Value=char(:, 1, SHARP)  OutDataTypeStr=uint8
  Column_1(1B) : Outport
  Column_2(1B) : Outport  Port=2
  Column_3(1B) : Outport  Port=3
  Column_4(1B) : Outport  Port=4
  Column_5(1B) : Outport  Port=5
  Column_6(1B) : Outport  Port=6
  Column_7(1B) : Outport  Port=7
  Column_8(1B) : Outport  Port=8
  wires:
  Byte_05/1 -> Column_6(1B)/1
  Byte_04/1 -> Column_5(1B)/1
  Byte_01/1 -> Column_2(1B)/1
  Byte_07/1 -> Column_8(1B)/1
  Byte_03/1 -> Column_4(1B)/1
  Byte_06/1 -> Column_7(1B)/1
  Byte_1/1 -> Column_1(1B)/1
  Byte_02/1 -> Column_3(1B)/1

== system unfinished_Test_Display/Character_Table/Characters(ARROW_DOWN..RECTANGLE)/Char_SPACE ==
  Byte_01 : Constant  Value=char(:, 2, SPACE)  OutDataTypeStr=uint8
  Byte_02 : Constant  Value=char(:, 3, SPACE)  OutDataTypeStr=uint8
  Byte_03 : Constant  Value=char(:, 4, SPACE)  OutDataTypeStr=uint8
  Byte_04 : Constant  Value=char(:, 5, SPACE)  OutDataTypeStr=uint8
  Byte_05 : Constant  Value=char(:, 6, SPACE)  OutDataTypeStr=uint8
  Byte_06 : Constant  Value=char(:, 7, SPACE)  OutDataTypeStr=uint8
  Byte_07 : Constant  Value=char(:, 8, SPACE)  OutDataTypeStr=uint8
  Byte_1 : Constant  Value=char(:, 1, SPACE)  OutDataTypeStr=uint8
  Column_1(1B) : Outport
  Column_2(1B) : Outport  Port=2
  Column_3(1B) : Outport  Port=3
  Column_4(1B) : Outport  Port=4
  Column_5(1B) : Outport  Port=5
  Column_6(1B) : Outport  Port=6
  Column_7(1B) : Outport  Port=7
  Column_8(1B) : Outport  Port=8
  wires:
  Byte_05/1 -> Column_6(1B)/1
  Byte_04/1 -> Column_5(1B)/1
  Byte_01/1 -> Column_2(1B)/1
  Byte_07/1 -> Column_8(1B)/1
  Byte_03/1 -> Column_4(1B)/1
  Byte_06/1 -> Column_7(1B)/1
  Byte_1/1 -> Column_1(1B)/1
  Byte_02/1 -> Column_3(1B)/1

== system unfinished_Test_Display/Character_Table/Characters(ARROW_DOWN..RECTANGLE)/Char_UNDERSCORE ==
  Byte_01 : Constant  Value=char(:, 2, UNDERSCORE)  OutDataTypeStr=uint8
  Byte_02 : Constant  Value=char(:, 3, UNDERSCORE)  OutDataTypeStr=uint8
  Byte_03 : Constant  Value=char(:, 4, UNDERSCORE)  OutDataTypeStr=uint8
  Byte_04 : Constant  Value=char(:, 5, UNDERSCORE)  OutDataTypeStr=uint8
  Byte_05 : Constant  Value=char(:, 6, UNDERSCORE)  OutDataTypeStr=uint8
  Byte_06 : Constant  Value=char(:, 7, UNDERSCORE)  OutDataTypeStr=uint8
  Byte_07 : Constant  Value=char(:, 8, UNDERSCORE)  OutDataTypeStr=uint8
  Byte_1 : Constant  Value=char(:, 1, UNDERSCORE)  OutDataTypeStr=uint8
  Column_1(1B) : Outport
  Column_2(1B) : Outport  Port=2
  Column_3(1B) : Outport  Port=3
  Column_4(1B) : Outport  Port=4
  Column_5(1B) : Outport  Port=5
  Column_6(1B) : Outport  Port=6
  Column_7(1B) : Outport  Port=7
  Column_8(1B) : Outport  Port=8
  wires:
  Byte_05/1 -> Column_6(1B)/1
  Byte_04/1 -> Column_5(1B)/1
  Byte_01/1 -> Column_2(1B)/1
  Byte_07/1 -> Column_8(1B)/1
  Byte_03/1 -> Column_4(1B)/1
  Byte_06/1 -> Column_7(1B)/1
  Byte_1/1 -> Column_1(1B)/1
  Byte_02/1 -> Column_3(1B)/1

== system unfinished_Test_Display/Character_Table/Characters(G..W)/Char_G ==
  Byte_01 : Constant  Value=char(:, 2, G)  OutDataTypeStr=uint8
  Byte_02 : Constant  Value=char(:, 3, G)  OutDataTypeStr=uint8
  Byte_03 : Constant  Value=char(:, 4, G)  OutDataTypeStr=uint8
  Byte_04 : Constant  Value=char(:, 5, G)  OutDataTypeStr=uint8
  Byte_05 : Constant  Value=char(:, 6, G)  OutDataTypeStr=uint8
  Byte_06 : Constant  Value=char(:, 7, G)  OutDataTypeStr=uint8
  Byte_07 : Constant  Value=char(:, 8, G)  OutDataTypeStr=uint8
  Byte_1 : Constant  Value=char(:, 1, G)  OutDataTypeStr=uint8
  Column_1(1B) : Outport
  Column_2(1B) : Outport  Port=2
  Column_3(1B) : Outport  Port=3
  Column_4(1B) : Outport  Port=4
  Column_5(1B) : Outport  Port=5
  Column_6(1B) : Outport  Port=6
  Column_7(1B) : Outport  Port=7
  Column_8(1B) : Outport  Port=8
  wires:
  Byte_05/1 -> Column_6(1B)/1
  Byte_04/1 -> Column_5(1B)/1
  Byte_01/1 -> Column_2(1B)/1
  Byte_07/1 -> Column_8(1B)/1
  Byte_03/1 -> Column_4(1B)/1
  Byte_06/1 -> Column_7(1B)/1
  Byte_1/1 -> Column_1(1B)/1
  Byte_02/1 -> Column_3(1B)/1

== system unfinished_Test_Display/Character_Table/Characters(G..W)/Char_H ==
  Byte_01 : Constant  Value=char(:, 2, H)  OutDataTypeStr=uint8
  Byte_02 : Constant  Value=char(:, 3, H)  OutDataTypeStr=uint8
  Byte_03 : Constant  Value=char(:, 4, H)  OutDataTypeStr=uint8
  Byte_04 : Constant  Value=char(:, 5, H)  OutDataTypeStr=uint8
  Byte_05 : Constant  Value=char(:, 6, H)  OutDataTypeStr=uint8
  Byte_06 : Constant  Value=char(:, 7, H)  OutDataTypeStr=uint8
  Byte_07 : Constant  Value=char(:, 8, H)  OutDataTypeStr=uint8
  Byte_1 : Constant  Value=char(:, 1, H)  OutDataTypeStr=uint8
  Column_1(1B) : Outport
  Column_2(1B) : Outport  Port=2
  Column_3(1B) : Outport  Port=3
  Column_4(1B) : Outport  Port=4
  Column_5(1B) : Outport  Port=5
  Column_6(1B) : Outport  Port=6
  Column_7(1B) : Outport  Port=7
  Column_8(1B) : Outport  Port=8
  wires:
  Byte_05/1 -> Column_6(1B)/1
  Byte_04/1 -> Column_5(1B)/1
  Byte_01/1 -> Column_2(1B)/1
  Byte_07/1 -> Column_8(1B)/1
  Byte_03/1 -> Column_4(1B)/1
  Byte_06/1 -> Column_7(1B)/1
  Byte_1/1 -> Column_1(1B)/1
  Byte_02/1 -> Column_3(1B)/1

== system unfinished_Test_Display/Character_Table/Characters(G..W)/Char_I ==
  Byte_01 : Constant  Value=char(:, 2, I)  OutDataTypeStr=uint8
  Byte_02 : Constant  Value=char(:, 3, I)  OutDataTypeStr=uint8
  Byte_03 : Constant  Value=char(:, 4, I)  OutDataTypeStr=uint8
  Byte_04 : Constant  Value=char(:, 5, I)  OutDataTypeStr=uint8
  Byte_05 : Constant  Value=char(:, 6, I)  OutDataTypeStr=uint8
  Byte_06 : Constant  Value=char(:, 7, I)  OutDataTypeStr=uint8
  Byte_07 : Constant  Value=char(:, 8, I)  OutDataTypeStr=uint8
  Byte_1 : Constant  Value=char(:, 1, I)  OutDataTypeStr=uint8
  Column_1(1B) : Outport
  Column_2(1B) : Outport  Port=2
  Column_3(1B) : Outport  Port=3
  Column_4(1B) : Outport  Port=4
  Column_5(1B) : Outport  Port=5
  Column_6(1B) : Outport  Port=6
  Column_7(1B) : Outport  Port=7
  Column_8(1B) : Outport  Port=8
  wires:
  Byte_05/1 -> Column_6(1B)/1
  Byte_04/1 -> Column_5(1B)/1
  Byte_01/1 -> Column_2(1B)/1
  Byte_07/1 -> Column_8(1B)/1
  Byte_03/1 -> Column_4(1B)/1
  Byte_06/1 -> Column_7(1B)/1
  Byte_1/1 -> Column_1(1B)/1
  Byte_02/1 -> Column_3(1B)/1

== system unfinished_Test_Display/Character_Table/Characters(G..W)/Char_J ==
  Byte_01 : Constant  Value=char(:, 2, J)  OutDataTypeStr=uint8
  Byte_02 : Constant  Value=char(:, 3, J)  OutDataTypeStr=uint8
  Byte_03 : Constant  Value=char(:, 4, J)  OutDataTypeStr=uint8
  Byte_04 : Constant  Value=char(:, 5, J)  OutDataTypeStr=uint8
  Byte_05 : Constant  Value=char(:, 6, J)  OutDataTypeStr=uint8
  Byte_06 : Constant  Value=char(:, 7, J)  OutDataTypeStr=uint8
  Byte_07 : Constant  Value=char(:, 8, J)  OutDataTypeStr=uint8
  Byte_1 : Constant  Value=char(:, 1, J)  OutDataTypeStr=uint8
  Column_1(1B) : Outport
  Column_2(1B) : Outport  Port=2
  Column_3(1B) : Outport  Port=3
  Column_4(1B) : Outport  Port=4
  Column_5(1B) : Outport  Port=5
  Column_6(1B) : Outport  Port=6
  Column_7(1B) : Outport  Port=7
  Column_8(1B) : Outport  Port=8
  wires:
  Byte_05/1 -> Column_6(1B)/1
  Byte_04/1 -> Column_5(1B)/1
  Byte_01/1 -> Column_2(1B)/1
  Byte_07/1 -> Column_8(1B)/1
  Byte_03/1 -> Column_4(1B)/1
  Byte_06/1 -> Column_7(1B)/1
  Byte_1/1 -> Column_1(1B)/1
  Byte_02/1 -> Column_3(1B)/1

== system unfinished_Test_Display/Character_Table/Characters(G..W)/Char_K ==
  Byte_01 : Constant  Value=char(:, 2, K)  OutDataTypeStr=uint8
  Byte_02 : Constant  Value=char(:, 3, K)  OutDataTypeStr=uint8
  Byte_03 : Constant  Value=char(:, 4, K)  OutDataTypeStr=uint8
  Byte_04 : Constant  Value=char(:, 5, K)  OutDataTypeStr=uint8
  Byte_05 : Constant  Value=char(:, 6, K)  OutDataTypeStr=uint8
  Byte_06 : Constant  Value=char(:, 7, K)  OutDataTypeStr=uint8
  Byte_07 : Constant  Value=char(:, 8, K)  OutDataTypeStr=uint8
  Byte_1 : Constant  Value=char(:, 1, K)  OutDataTypeStr=uint8
  Column_1(1B) : Outport
  Column_2(1B) : Outport  Port=2
  Column_3(1B) : Outport  Port=3
  Column_4(1B) : Outport  Port=4
  Column_5(1B) : Outport  Port=5
  Column_6(1B) : Outport  Port=6
  Column_7(1B) : Outport  Port=7
  Column_8(1B) : Outport  Port=8
  wires:
  Byte_05/1 -> Column_6(1B)/1
  Byte_04/1 -> Column_5(1B)/1
  Byte_01/1 -> Column_2(1B)/1
  Byte_07/1 -> Column_8(1B)/1
  Byte_03/1 -> Column_4(1B)/1
  Byte_06/1 -> Column_7(1B)/1
  Byte_1/1 -> Column_1(1B)/1
  Byte_02/1 -> Column_3(1B)/1

== system unfinished_Test_Display/Character_Table/Characters(G..W)/Char_L ==
  Byte_01 : Constant  Value=char(:, 2, L)  OutDataTypeStr=uint8
  Byte_02 : Constant  Value=char(:, 3, L)  OutDataTypeStr=uint8
  Byte_03 : Constant  Value=char(:, 4, L)  OutDataTypeStr=uint8
  Byte_04 : Constant  Value=char(:, 5, L)  OutDataTypeStr=uint8
  Byte_05 : Constant  Value=char(:, 6, L)  OutDataTypeStr=uint8
  Byte_06 : Constant  Value=char(:, 7, L)  OutDataTypeStr=uint8
  Byte_07 : Constant  Value=char(:, 8, L)  OutDataTypeStr=uint8
  Byte_1 : Constant  Value=char(:, 1, L)  OutDataTypeStr=uint8
  Column_1(1B) : Outport
  Column_2(1B) : Outport  Port=2
  Column_3(1B) : Outport  Port=3
  Column_4(1B) : Outport  Port=4
  Column_5(1B) : Outport  Port=5
  Column_6(1B) : Outport  Port=6
  Column_7(1B) : Outport  Port=7
  Column_8(1B) : Outport  Port=8
  wires:
  Byte_05/1 -> Column_6(1B)/1
  Byte_04/1 -> Column_5(1B)/1
  Byte_01/1 -> Column_2(1B)/1
  Byte_07/1 -> Column_8(1B)/1
  Byte_03/1 -> Column_4(1B)/1
  Byte_06/1 -> Column_7(1B)/1
  Byte_1/1 -> Column_1(1B)/1
  Byte_02/1 -> Column_3(1B)/1

== system unfinished_Test_Display/Character_Table/Characters(G..W)/Char_M ==
  Byte_01 : Constant  Value=char(:, 2, M)  OutDataTypeStr=uint8
  Byte_02 : Constant  Value=char(:, 3, M)  OutDataTypeStr=uint8
  Byte_03 : Constant  Value=char(:, 4, M)  OutDataTypeStr=uint8
  Byte_04 : Constant  Value=char(:, 5, M)  OutDataTypeStr=uint8
  Byte_05 : Constant  Value=char(:, 6, M)  OutDataTypeStr=uint8
  Byte_06 : Constant  Value=char(:, 7, M)  OutDataTypeStr=uint8
  Byte_07 : Constant  Value=char(:, 8, M)  OutDataTypeStr=uint8
  Byte_1 : Constant  Value=char(:, 1, M)  OutDataTypeStr=uint8
  Column_1(1B) : Outport
  Column_2(1B) : Outport  Port=2
  Column_3(1B) : Outport  Port=3
  Column_4(1B) : Outport  Port=4
  Column_5(1B) : Outport  Port=5
  Column_6(1B) : Outport  Port=6
  Column_7(1B) : Outport  Port=7
  Column_8(1B) : Outport  Port=8
  wires:
  Byte_05/1 -> Column_6(1B)/1
  Byte_04/1 -> Column_5(1B)/1
  Byte_01/1 -> Column_2(1B)/1
  Byte_07/1 -> Column_8(1B)/1
  Byte_03/1 -> Column_4(1B)/1
  Byte_06/1 -> Column_7(1B)/1
  Byte_1/1 -> Column_1(1B)/1
  Byte_02/1 -> Column_3(1B)/1

== system unfinished_Test_Display/Character_Table/Characters(G..W)/Char_N ==
  Byte_01 : Constant  Value=char(:, 2, N)  OutDataTypeStr=uint8
  Byte_02 : Constant  Value=char(:, 3, N)  OutDataTypeStr=uint8
  Byte_03 : Constant  Value=char(:, 4, N)  OutDataTypeStr=uint8
  Byte_04 : Constant  Value=char(:, 5, N)  OutDataTypeStr=uint8
  Byte_05 : Constant  Value=char(:, 6, N)  OutDataTypeStr=uint8
  Byte_06 : Constant  Value=char(:, 7, N)  OutDataTypeStr=uint8
  Byte_07 : Constant  Value=char(:, 8, N)  OutDataTypeStr=uint8
  Byte_1 : Constant  Value=char(:, 1, N)  OutDataTypeStr=uint8
  Column_1(1B) : Outport
  Column_2(1B) : Outport  Port=2
  Column_3(1B) : Outport  Port=3
  Column_4(1B) : Outport  Port=4
  Column_5(1B) : Outport  Port=5
  Column_6(1B) : Outport  Port=6
  Column_7(1B) : Outport  Port=7
  Column_8(1B) : Outport  Port=8
  wires:
  Byte_05/1 -> Column_6(1B)/1
  Byte_04/1 -> Column_5(1B)/1
  Byte_01/1 -> Column_2(1B)/1
  Byte_07/1 -> Column_8(1B)/1
  Byte_03/1 -> Column_4(1B)/1
  Byte_06/1 -> Column_7(1B)/1
  Byte_1/1 -> Column_1(1B)/1
  Byte_02/1 -> Column_3(1B)/1

== system unfinished_Test_Display/Character_Table/Characters(G..W)/Char_O ==
  Byte_01 : Constant  Value=char(:, 2, O)  OutDataTypeStr=uint8
  Byte_02 : Constant  Value=char(:, 3, O)  OutDataTypeStr=uint8
  Byte_03 : Constant  Value=char(:, 4, O)  OutDataTypeStr=uint8
  Byte_04 : Constant  Value=char(:, 5, O)  OutDataTypeStr=uint8
  Byte_05 : Constant  Value=char(:, 6, O)  OutDataTypeStr=uint8
  Byte_06 : Constant  Value=char(:, 7, O)  OutDataTypeStr=uint8
  Byte_07 : Constant  Value=char(:, 8, O)  OutDataTypeStr=uint8
  Byte_1 : Constant  Value=char(:, 1, O)  OutDataTypeStr=uint8
  Column_1(1B) : Outport
  Column_2(1B) : Outport  Port=2
  Column_3(1B) : Outport  Port=3
  Column_4(1B) : Outport  Port=4
  Column_5(1B) : Outport  Port=5
  Column_6(1B) : Outport  Port=6
  Column_7(1B) : Outport  Port=7
  Column_8(1B) : Outport  Port=8
  wires:
  Byte_05/1 -> Column_6(1B)/1
  Byte_04/1 -> Column_5(1B)/1
  Byte_01/1 -> Column_2(1B)/1
  Byte_07/1 -> Column_8(1B)/1
  Byte_03/1 -> Column_4(1B)/1
  Byte_06/1 -> Column_7(1B)/1
  Byte_1/1 -> Column_1(1B)/1
  Byte_02/1 -> Column_3(1B)/1

== system unfinished_Test_Display/Character_Table/Characters(G..W)/Char_P ==
  Byte_01 : Constant  Value=char(:, 2, P)  OutDataTypeStr=uint8
  Byte_02 : Constant  Value=char(:, 3, P)  OutDataTypeStr=uint8
  Byte_03 : Constant  Value=char(:, 4, P)  OutDataTypeStr=uint8
  Byte_04 : Constant  Value=char(:, 5, P)  OutDataTypeStr=uint8
  Byte_05 : Constant  Value=char(:, 6, P)  OutDataTypeStr=uint8
  Byte_06 : Constant  Value=char(:, 7, P)  OutDataTypeStr=uint8
  Byte_07 : Constant  Value=char(:, 8, P)  OutDataTypeStr=uint8
  Byte_1 : Constant  Value=char(:, 1, P)  OutDataTypeStr=uint8
  Column_1(1B) : Outport
  Column_2(1B) : Outport  Port=2
  Column_3(1B) : Outport  Port=3
  Column_4(1B) : Outport  Port=4
  Column_5(1B) : Outport  Port=5
  Column_6(1B) : Outport  Port=6
  Column_7(1B) : Outport  Port=7
  Column_8(1B) : Outport  Port=8
  wires:
  Byte_05/1 -> Column_6(1B)/1
  Byte_04/1 -> Column_5(1B)/1
  Byte_01/1 -> Column_2(1B)/1
  Byte_07/1 -> Column_8(1B)/1
  Byte_03/1 -> Column_4(1B)/1
  Byte_06/1 -> Column_7(1B)/1
  Byte_1/1 -> Column_1(1B)/1
  Byte_02/1 -> Column_3(1B)/1

== system unfinished_Test_Display/Character_Table/Characters(G..W)/Char_R ==
  Byte_01 : Constant  Value=char(:, 2, R)  OutDataTypeStr=uint8
  Byte_02 : Constant  Value=char(:, 3, R)  OutDataTypeStr=uint8
  Byte_03 : Constant  Value=char(:, 4, R)  OutDataTypeStr=uint8
  Byte_04 : Constant  Value=char(:, 5, R)  OutDataTypeStr=uint8
  Byte_05 : Constant  Value=char(:, 6, R)  OutDataTypeStr=uint8
  Byte_06 : Constant  Value=char(:, 7, R)  OutDataTypeStr=uint8
  Byte_07 : Constant  Value=char(:, 8, R)  OutDataTypeStr=uint8
  Byte_1 : Constant  Value=char(:, 1, R)  OutDataTypeStr=uint8
  Column_1(1B) : Outport
  Column_2(1B) : Outport  Port=2
  Column_3(1B) : Outport  Port=3
  Column_4(1B) : Outport  Port=4
  Column_5(1B) : Outport  Port=5
  Column_6(1B) : Outport  Port=6
  Column_7(1B) : Outport  Port=7
  Column_8(1B) : Outport  Port=8
  wires:
  Byte_05/1 -> Column_6(1B)/1
  Byte_04/1 -> Column_5(1B)/1
  Byte_01/1 -> Column_2(1B)/1
  Byte_07/1 -> Column_8(1B)/1
  Byte_03/1 -> Column_4(1B)/1
  Byte_06/1 -> Column_7(1B)/1
  Byte_1/1 -> Column_1(1B)/1
  Byte_02/1 -> Column_3(1B)/1

== system unfinished_Test_Display/Character_Table/Characters(G..W)/Char_S ==
  Byte_01 : Constant  Value=char(:, 2, S)  OutDataTypeStr=uint8
  Byte_02 : Constant  Value=char(:, 3, S)  OutDataTypeStr=uint8
  Byte_03 : Constant  Value=char(:, 4, S)  OutDataTypeStr=uint8
  Byte_04 : Constant  Value=char(:, 5, S)  OutDataTypeStr=uint8
  Byte_05 : Constant  Value=char(:, 6, S)  OutDataTypeStr=uint8
  Byte_06 : Constant  Value=char(:, 7, S)  OutDataTypeStr=uint8
  Byte_07 : Constant  Value=char(:, 8, S)  OutDataTypeStr=uint8
  Byte_1 : Constant  Value=char(:, 1, S)  OutDataTypeStr=uint8
  Column_1(1B) : Outport
  Column_2(1B) : Outport  Port=2
  Column_3(1B) : Outport  Port=3
  Column_4(1B) : Outport  Port=4
  Column_5(1B) : Outport  Port=5
  Column_6(1B) : Outport  Port=6
  Column_7(1B) : Outport  Port=7
  Column_8(1B) : Outport  Port=8
  wires:
  Byte_05/1 -> Column_6(1B)/1
  Byte_04/1 -> Column_5(1B)/1
  Byte_01/1 -> Column_2(1B)/1
  Byte_07/1 -> Column_8(1B)/1
  Byte_03/1 -> Column_4(1B)/1
  Byte_06/1 -> Column_7(1B)/1
  Byte_1/1 -> Column_1(1B)/1
  Byte_02/1 -> Column_3(1B)/1

== system unfinished_Test_Display/Character_Table/Characters(G..W)/Char_T ==
  Byte_01 : Constant  Value=char(:, 2, T)  OutDataTypeStr=uint8
  Byte_02 : Constant  Value=char(:, 3, T)  OutDataTypeStr=uint8
  Byte_03 : Constant  Value=char(:, 4, T)  OutDataTypeStr=uint8
  Byte_04 : Constant  Value=char(:, 5, T)  OutDataTypeStr=uint8
  Byte_05 : Constant  Value=char(:, 6, T)  OutDataTypeStr=uint8
  Byte_06 : Constant  Value=char(:, 7, T)  OutDataTypeStr=uint8
  Byte_07 : Constant  Value=char(:, 8, T)  OutDataTypeStr=uint8
  Byte_1 : Constant  Value=char(:, 1, T)  OutDataTypeStr=uint8
  Column_1(1B) : Outport
  Column_2(1B) : Outport  Port=2
  Column_3(1B) : Outport  Port=3
  Column_4(1B) : Outport  Port=4
  Column_5(1B) : Outport  Port=5
  Column_6(1B) : Outport  Port=6
  Column_7(1B) : Outport  Port=7
  Column_8(1B) : Outport  Port=8
  wires:
  Byte_05/1 -> Column_6(1B)/1
  Byte_04/1 -> Column_5(1B)/1
  Byte_01/1 -> Column_2(1B)/1
  Byte_07/1 -> Column_8(1B)/1
  Byte_03/1 -> Column_4(1B)/1
  Byte_06/1 -> Column_7(1B)/1
  Byte_1/1 -> Column_1(1B)/1
  Byte_02/1 -> Column_3(1B)/1
